simulink model "model"  (R2024a)
settings: Solver=VariableStepAuto  StartTime=0.0  StopTime=10.0  RelTol=1e-3
settings Model: Creator=eva  LastModifiedBy=eva

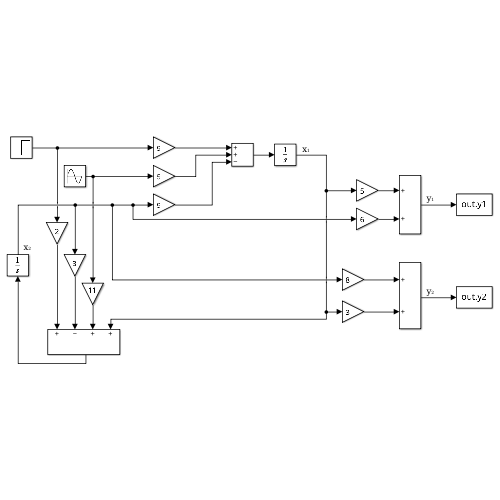
[thumbnail: Simulink's stored preview of the top-level diagram]
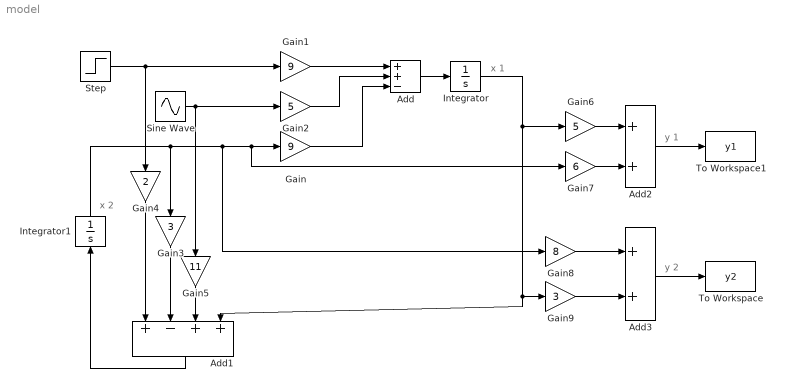
== system model ==
  note: x 1
  note: x 2
  note: y 1
  note: y 2
  Add : Sum  Inputs=++-
  Add1 : Sum  Inputs=+-++
  Add2 : Sum
  Add3 : Sum
  Gain : Gain  Gain=9
  Gain1 : Gain  Gain=9
  Gain2 : Gain  Gain=5
  Gain3 : Gain  Gain=3
  Gain4 : Gain  Gain=2
  Gain5 : Gain  Gain=11
  Gain6 : Gain  Gain=5
  Gain7 : Gain  Gain=6
  Gain8 : Gain  Gain=8
  Gain9 : Gain  Gain=3
  Integrator : Integrator
  Integrator1 : Integrator
  Sine Wave : Sin  SampleTime=0
  Step : Step  SampleTime=0
  To Workspace : ToWorkspace  VariableName=y2  SaveFormat=Timeseries  SampleTime=-1
  To Workspace1 : ToWorkspace  VariableName=y1  SaveFormat=Timeseries  SampleTime=-1
  wires:
  Step/1 -> Gain1/1, Gain4/1
  Integrator/1 -> Add1/4, Gain9/1, Gain6/1
  Integrator1/1 -> Gain/1, Gain7/1, Gain8/1, Gain3/1
  Gain/1 -> Add/3
  Gain1/1 -> Add/1
  Gain2/1 -> Add/2
  Add/1 -> Integrator/1
  Sine Wave/1 -> Gain2/1, Gain5/1
  Add1/1 -> Integrator1/1
  Gain6/1 -> Add2/1
  Gain7/1 -> Add2/2
  Add2/1 -> To Workspace1/1
  Add3/1 -> To Workspace/1
  Gain4/1 -> Add1/1
  Gain3/1 -> Add1/2
  Gain5/1 -> Add1/3
  Gain8/1 -> Add3/1
  Gain9/1 -> Add3/2
